simulink model "solar_tracking_with_PIDcontrol"  (R2024b)
settings: Solver=VariableStepAuto  StartTime=-5  StopTime=30  RelTol=1e-3
model workspace (MAT data in the model file):
  J = 8.6
  Kd = 5
  Kf = 0.07
  Kg = 2000
  Kt = 0.07
  L = 1e-05
  R = 10
libraries: slpidlib x1
settings Model: Creator=haider  LastModifiedBy=Luke
settings SolverCC: AlgebraicLoopSolver=TrustRegion
settings DebuggingCC: UnconnectedInputMsg=warning  UnconnectedOutputMsg=warning  UnconnectedLineMsg=warning
settings ModelReferenceCC: EnableRefExpFcnMdlSchedulingChecks=on
settings RTWCC: GPUComputeCapability=3.5  DLArmComputeVersion=19.05

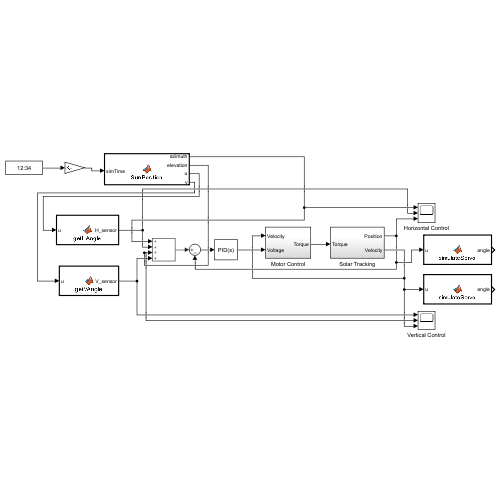
[thumbnail: Simulink's stored preview of the top-level diagram]
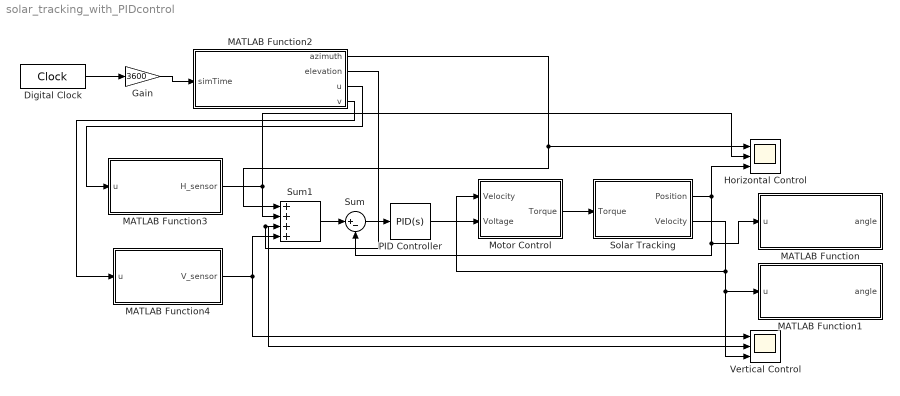
== system solar_tracking_with_PIDcontrol ==
  Digital Clock : DigitalClock
  Gain : Gain  Gain=3600
  "Horizontal Control " : Scope  NumInputPorts=3
  MATLAB Function : MATLAB Function  TreatAsAtomicUnit=on
  MATLAB Function1 : MATLAB Function  TreatAsAtomicUnit=on
  MATLAB Function2 : MATLAB Function  TreatAsAtomicUnit=on
  MATLAB Function3 : MATLAB Function  TreatAsAtomicUnit=on
  MATLAB Function4 : MATLAB Function  TreatAsAtomicUnit=on
  Motor Control : Subsystem
  PID Controller : slpidlib/PID Controller  Controller=PID  Form=Parallel  TimeDomain=Continuous-time  UseExternalTs=off  SampleTime=-1  IntegratorMethod=Forward Euler  FilterMethod=Forward Euler  ControllerParametersSource=internal  P=320.814393277  I=600.49625354  UseKiTs=off  D=-36.7846486438784  UseExternalDerivativeSource=off  N=8.58758696842  UseFilter=on  TunerSelectOption=Transfer Function Based (PID Tuner App)  InitialConditionSource=internal  InitialConditionForIntegrator=0  InitialConditionForFilter=0  DifferentiatorICPrevScaledInput=0  ExternalReset=none  TrackingMode=off  Kt=1  LimitOutput=off  SatLimitsSource=internal  UpperSaturationLimit=inf  LowerSaturationLimit=-inf  LinearizeAsGain=on  AntiWindupMode=none  Kb=1  LimitIntegrator=off  UpperIntegratorSaturationLimit=inf  LowerIntegratorSaturationLimit=-inf  POutMin=[]  POutMax=[]  IOutMin=[]  IOutMax=[]  DOutMin=[]  DOutMax=[]  NOutMin=[]  NOutMax=[]  SumOutMin=[]  SumOutMax=[]  SaturationOutMin=[]  SaturationOutMax=[]  PParamMin=[]  PParamMax=[]  IParamMin=[]  IParamMax=[]  DParamMin=[]  DParamMax=[]  NParamMin=[]  NParamMax=[]  KbParamMin=[]  KbParamMax=[]  KtParamMin=[]  KtParamMax=[]  KbOutMin=[]  KbOutMax=[]  KtOutMin=[]  KtOutMax=[]  IntegratorOutMin=[]  IntegratorOutMax=[]  FilterOutMin=[]  FilterOutMax=[]  SumI1OutMin=[]  SumI1OutMax=[]  SumI2OutMin=[]  SumI2OutMax=[]  SumI3OutMin=[]  SumI3OutMax=[]  SumI4OutMin=[]  SumI4OutMax=[]  SumDOutMin=[]  SumDOutMax=[]  DifferentiatorOutMin=[]  DifferentiatorOutMax=[]  FilterDiffOutCoefMin=[]  FilterDiffOutCoefMax=[]  ReciprocalOutMin=[]  ReciprocalOutMax=[]  SumDenOutMin=[]  SumDenOutMax=[]  SumNumOutMin=[]  SumNumOutMax=[]  DivideOutMin=[]  DivideOutMax=[]  UdiffTsProdOutMin=[]  UdiffTsProdOutMax=[]  NTsProdOutMin=[]  NTsProdOutMax=[]  UintegralTsProdOutMin=[]  UintegralTsProdOutMax=[]  UngainTsProdOutMin=[]  UngainTsProdOutMax=[]  ClampingZeroOutDataTypeStr=Inherit: Inherit via back propagation  ClampingZeroOutMin=[]  ClampingZeroOutMax=[]  FilterDenConstantOutDataTypeStr=Inherit: Inherit via back propagation  FilterDenConstantOutMin=[]  FilterDenConstantOutMax=[]  PCopyOutDataTypeStr=Inherit: Inherit via back propagation  PCopyOutMin=[]  PCopyOutMax=[]  NCopyOutDataTypeStr=Inherit: Inherit via back propagation  NCopyOutMin=[]  NCopyOutMax=[]  IntegratorContinuousStateAttributes=''  IntegratorStateMustResolveToSignalObject=off  IntegratorRTWStateStorageClass=Auto  FilterContinuousStateAttributes=''  FilterStateMustResolveToSignalObject=off  FilterRTWStateStorageClass=Auto  ParallelPVariant=InternalParameters  IdealPVariant=Disabled  IVariant=InternalParameters  DVariant=InternalParameters  IntegratorVariant=Continuous  SatVariant=Disabled  AWVariant=Passthrough  PCopyVariant=Disabled  TRVariant=Disabled  FdbkBlocksVariant=Forward  IdealPFdbkVariant=Disabled  SatFdbkVariant=Disabled  DerivativeFilterVariant=ContFilter  NVariant=InternalParameters  NCopyVariant=Disabled  FilterICVariant=InternalICsFilter  IntegratorICVariant=InternalICs  ExternalResetVariant=Disabled  TRSumVariant=Passthrough  SumFdbkVariant=Disabled  SumVariant=Sum_PID  TsampFilterVariant=InternalTs  TsampNgainVariant=Passthrough  TsampIntegralVariant=Disabled_SignalSpec  ExternalSaturationOutDataTypeStr=Inherit: Same as second input  DerivativeSourceVariant=ErrorSignal  PreIntVariant=InternalPreInt
  Solar Tracking : Subsystem
  Sum : Sum  Inputs=|+-
  Sum1 : Sum  Inputs=+|+|+|+
  "Vertical Control " : Scope  NumInputPorts=3
  wires:
  Solar Tracking/1(Position) -> MATLAB Function/1(u), Sum/2, "Horizontal Control "/3
  PID Controller/1 -> Motor Control/2(Voltage)
  Motor Control/1(Torque) -> Solar Tracking/1("Torque ")
  Sum/1 -> PID Controller/1
  Sum1/1 -> Sum/1
  Solar Tracking/2(Velocity) -> Motor Control/1(Velocity), "Vertical Control "/3, MATLAB Function1/1(u)
  Gain/1 -> MATLAB Function2/1(simTime)
  Digital Clock/1 -> Gain/1
  MATLAB Function2/1(azimuth) -> Sum1/1, "Horizontal Control "/1
  MATLAB Function2/2(elevation) -> "Vertical Control "/2, Sum1/3
  MATLAB Function3/1(H_sensor) -> "Horizontal Control "/2, Sum1/2
  MATLAB Function4/1(V_sensor) -> "Vertical Control "/1, Sum1/4
  MATLAB Function2/3(u) -> MATLAB Function3/1(u)
  MATLAB Function2/4(v) -> MATLAB Function4/1(u)

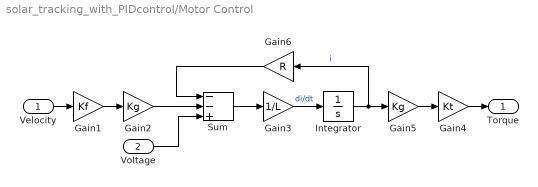
== system solar_tracking_with_PIDcontrol/Motor Control ==
  Velocity : Inport
  Voltage : Inport  Port=2
  Gain1 : Gain  Gain=Kf
  Gain2 : Gain  Gain=Kg
  Gain3 : Gain  Gain=1/L
  Gain4 : Gain  Gain=Kt
  Gain5 : Gain  Gain=Kg
  Gain6 : Gain  Gain=R
  Integrator : Integrator
  Sum : Sum  Inputs=-|-|+
  Torque : Outport
  wires:
  Integrator/1 -> Gain5/1, Gain6/1  "i"
  Velocity/1 -> Gain1/1
  Gain1/1 -> Gain2/1
  Sum/1 -> Gain3/1
  Gain3/1 -> Integrator/1  "di/dt"
  Gain5/1 -> Gain4/1
  Gain4/1 -> Torque/1
  Gain6/1 -> Sum/1
  Gain2/1 -> Sum/2
  Voltage/1 -> Sum/3

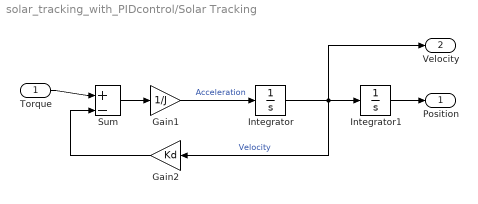
== system solar_tracking_with_PIDcontrol/Solar Tracking ==
  "Torque " : Inport
  Gain1 : Gain  Gain=1/J
  Gain2 : Gain  Gain=Kd
  Integrator : Integrator
  Integrator1 : Integrator
  Sum : Sum  Inputs=+|-
  Position : Outport
  Velocity : Outport  Port=2
  wires:
  Integrator/1 -> Gain2/1, Velocity/1, Integrator1/1  "Velocity"
  Sum/1 -> Gain1/1
  Gain2/1 -> Sum/2
  "Torque "/1 -> Sum/1
  Integrator1/1 -> Position/1
  Gain1/1 -> Integrator/1  "Acceleration"

== matlab function solar_tracking_with_PIDcontrol/MATLAB Function1 ==
  settings: updateMethod=DISCRETE
  data: u input; angle output
function angle = simulateServo(u)
% u: input torque (PID output)
% Simple simulation of servo movement using gain and clamping

persistent theta;
if isempty(theta)
    theta = 90; % initial position at 90 degrees
end

% Parameters
K = 0.1;  % responsiveness gain
dt = 0.01; % simulation time step (s)

% Simulate angle update
theta = theta + K * u * dt;

% Clamp angle between 0 and 180
theta = min(max(theta, 0), 180);

% Output
angle = theta;
end

== matlab function solar_tracking_with_PIDcontrol/MATLAB Function ==
  settings: updateMethod=DISCRETE
  data: u input; angle output
function angle = simulateServo(u)
% u: input torque (PID output)
% Simple simulation of servo movement using gain and clamping

persistent theta;
if isempty(theta)
    theta = 90; % initial position at 90 degrees
end

% Parameters
K = 0.1;  % responsiveness gain
dt = 0.01; % simulation time step (s)

% Simulate angle update
theta = theta + K * u * dt;

% Clamp angle between 0 and 180
theta = min(max(theta, 0), 180);

% Output
angle = theta;
end

== matlab function solar_tracking_with_PIDcontrol/MATLAB Function2 ==
  data: simTime input; azimuth output; elevation output; u output; v output
function [azimuth, elevation, u, v] = SunPosition(simTime)
% Inputs:
%   simTime - Time in seconds since Jan 1, 00:00:00
% Outputs:
%   azimuth, elevation - Sun's position angles in degrees
%   u, v - direction cosines representing sun's horizontal and vertical projections

% --- Constants ---
latitude = 12.91;    % Mangalore, India
longitude = 74.85;
UTC_offset = 5.5;    % IST

% --- Time Calculations ---
secs_per_day = 86400;
dayOfYear = floor(simTime / secs_per_day) + 1;
secondsToday = mod(simTime, secs_per_day);

% Time in UTC hours (decimal)
timeUTC = (secondsToday / 3600) - UTC_offset;

% --- Declination ---
decl = 23.45 * sind(360 * (284 + dayOfYear) / 365);

% --- Equation of Time ---
B = 360 * (dayOfYear - 81) / 364;
EoT = 9.87 * sind(2*B) - 7.53 * cosd(B) - 1.5 * sind(B); % in minutes

% --- Time Correction ---
TC = 4 * (longitude - 15 * round(longitude/15)) + EoT;  % in minutes

% --- Local Solar Time (LST) ---
LST = timeUTC + TC / 60; % decimal hours

% --- Hour angle ---
hourAngle = 15 * (LST - 12);

% --- Convert to radians ---
latRad = deg2rad(latitude);
declRad = deg2rad(decl);
haRad = deg2rad(hourAngle);

% --- Elevation angle ---
elevation = asind(sin(latRad)*sin(declRad) + cos(latRad)*cos(declRad)*cos(haRad));

% --- Azimuth angle ---
cosAz = (sin(declRad) - sin(latRad)*sind(elevation)) / (cos(latRad)*cosd(elevation));
% Clamp to [-1, 1] to avoid domain errors
cosAz = max(min(cosAz, 1), -1);
azimuth = acosd(cosAz);

% Adjust azimuth for morning/afternoon
if hourAngle > 0
    azimuth = 360 - azimuth;
end

% --- Calculate u and v ---
% Convert azimuth and elevation to radians for trig functions
azRad = deg2rad(azimuth);
elRad = deg2rad(elevation);

% u and v as horizontal and vertical direction cosines
u = cos(elRad) * cos(azRad);
v = cos(elRad) * sin(azRad);

end

== matlab function solar_tracking_with_PIDcontrol/MATLAB Function3 ==
  data: u input; H_sensor output
function H_sensor = getHAngle(u)
% Simulated horizontal sensor reading
% u = current angle from horizontal servo

% Just pass through or add noise if needed
H_sensor = u;

% Optional: add simulated sensor noise
% noise = 0.5 * randn(); % small Gaussian noise
% H_sensor = u + noise;
end

== matlab function solar_tracking_with_PIDcontrol/MATLAB Function4 ==
  data: u input; V_sensor output
function V_sensor = getVAngle(u)
% Simulated vertical sensor reading
% u = current angle from vertical servo

V_sensor = u;

% Optional: add sensor noise
% noise = 0.5 * randn(); % small Gaussian noise
% V_sensor = u + noise;
end
